simulink model "Monza_borroso"  (R2021b)
settings: Solver=VariableStepAuto  StartTime=0.0  StopTime=tsim  RelTol=1e-3
values from neighbouring files (symbols this model uses):
  dificultad = 4    [ControlBorroso.m]    (also in GA.m)
  FSetDError = FuzzySet(reglasDErrorF{:})    [ControlBorroso.m]    (also in GA.m)
  FSetError = FuzzySet(reglasErrorF{:})    [ControlBorroso.m]    (also in GA.m)
  LUT = [ind(1)   ind(2)   ind(3)  ind(4)  -ind(12) ... (first row only)    [ControlBorroso.m]    (also in GA.m; LUT_GA.mat = [0.476090111801 -0.0536947834317 0.322270109538 0.2576074503)
  Ts = 0.033    [ControlBorroso.m]    (also in GA.m)
undefined symbols (not defined in the file or in its folder): ControlBorrosoErrorLUT
libraries: simulink x1
settings Model: Creator=christian  LastModifiedBy=pablo
settings SolverCC: AlgebraicLoopSolver=TrustRegion
settings DataIOCC: ReturnWorkspaceOutputs=off
settings DebuggingCC: SFMachineParentedDataDiag=warning  ArithmeticOperatorsInVariantConditions=warning
settings SFSimCC: SimUseLocalCustomCode=off  CustomCodeUndefinedFunction=UseInterfaceOnly
settings RTWCC: RTWUseLocalCustomCode=off

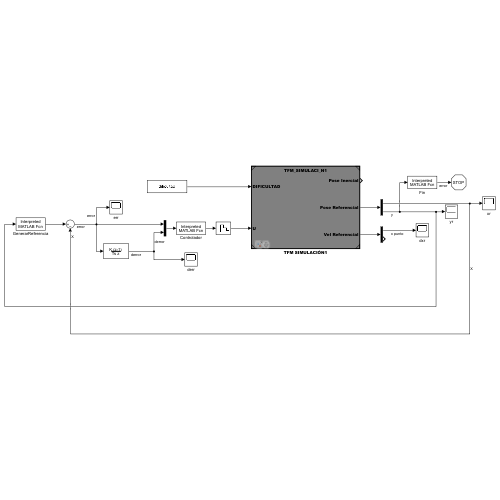
[thumbnail: Simulink's stored preview of the top-level diagram]
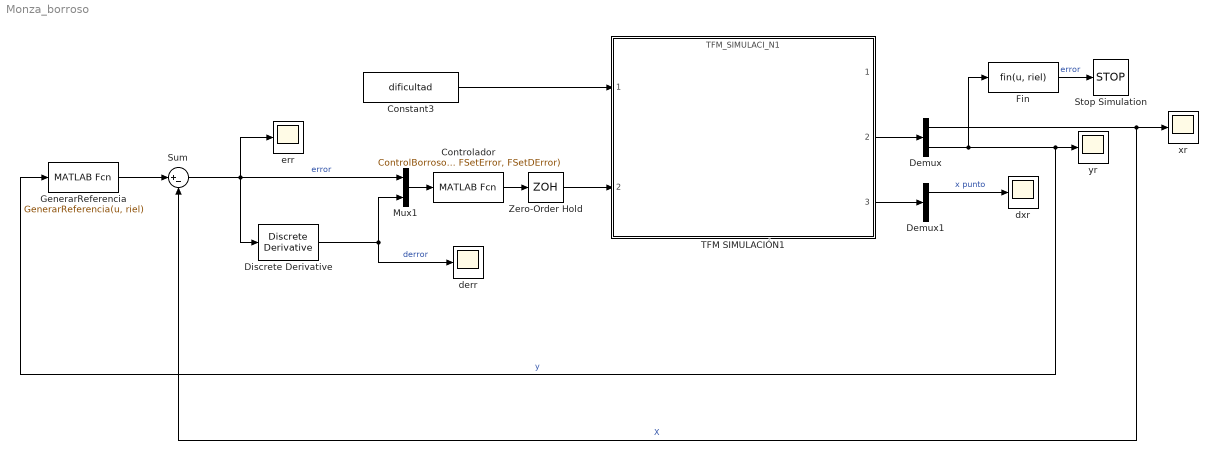
== system Monza_borroso ==
  Constant3 : Constant  Value=dificultad
  Controlador : MATLABFcn  MATLABFcn=ControlBorrosoErrorLUT(u(1), u(2), LUT, FSetError, FSetDError)  OutputDimensions=1
  Demux : Demux  Outputs=2
  Demux1 : Demux  Outputs=2
  Discrete Derivative : simulink/Discrete/Discrete Derivative  gainval=1  ICPrevScaledInput=0.0  OutMin=[]  OutMax=[]  OutDataType=fixdt(1, 16)  OutScaling=2^-10  DoSatur=off
  Fin : MATLABFcn  MATLABFcn=fin(u, riel)  OutputDimensions=1
  GenerarReferencia : MATLABFcn  MATLABFcn=GenerarReferencia(u, riel)
  Mux1 : Mux  Inputs=2
  Stop Simulation : Stop
  Sum : Sum  Inputs=|+-
  TFM SIMULACIÓN1 : ModelReference  ModelNameDialog=TFM_SIMULACI_N1.slx  UsingDefaultArgumentValue=0,0  SimulationMode=Normal  ModelReferenceVersion=9.1  Gain=0.05  Gain2=0.0223  SimulationMode=Normal
  Zero-Order Hold : ZeroOrderHold  SampleTime=Ts
  derr : Scope
  dxr : Scope
  err : Scope
  xr : Scope
  yr : Scope
  wires:
  Constant3/1 -> TFM SIMULACIÓN1/1
  TFM SIMULACIÓN1/2 -> Demux/1
  TFM SIMULACIÓN1/3 -> Demux1/1
  Demux1/1 -> dxr/1  "x punto"
  Demux/1 -> Sum/2, xr/1  "X"
  Discrete Derivative/1 -> Mux1/2, derr/1  "derror"
  Mux1/1 -> Controlador/1
  GenerarReferencia/1 -> Sum/1
  Demux/2 -> GenerarReferencia/1, yr/1, Fin/1  "y"
  Fin/1 -> Stop Simulation/1  "error"
  Sum/1 -> Discrete Derivative/1, err/1, Mux1/1  "error"
  Controlador/1 -> Zero-Order Hold/1
  Zero-Order Hold/1 -> TFM SIMULACIÓN1/2
